simulink model "Plant"  (R2021a)
settings: Solver=ode8  StartTime=0.0  StopTime=20  FixedStep=0.0001  RelTol=1e-3
model workspace (MAT data in the model file):
  initial_current = 0
undefined symbols (not defined in the file): DiscIntNeverNeededParam
settings Model: Creator=zhaoh  LastModifiedBy=zhaoh

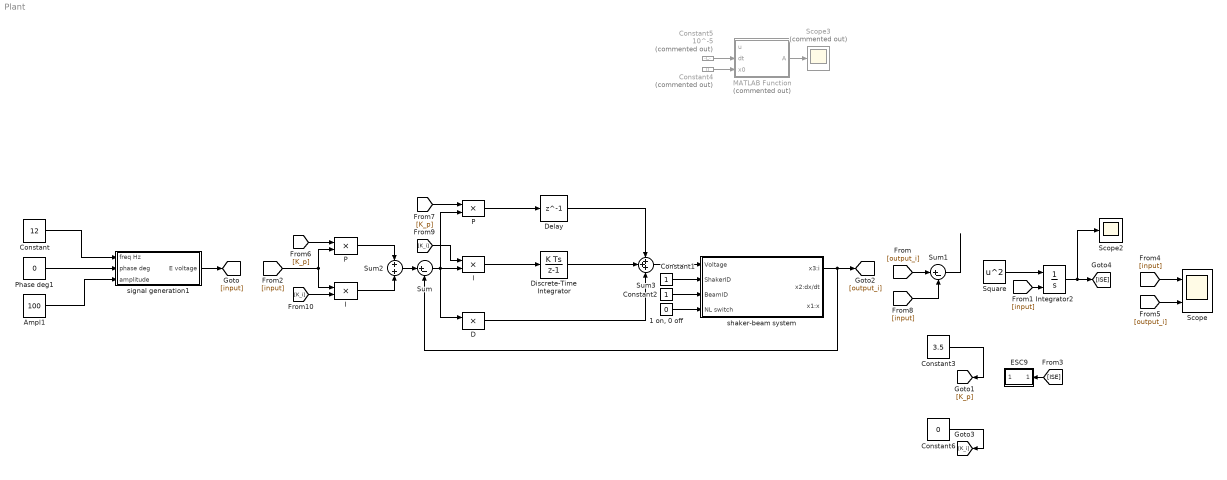
== system Plant ==
  "1 on, 0 off" : Constant  Value=0
  Ampl1 : Constant  Value=100
  Constant : Constant  Value=12
  Constant1 : Constant
  Constant2 : Constant
  Constant3 : Constant  Value=3.5
  Constant4 : Constant  Commented=on  Value=0
  Constant5 : Constant  Commented=on  Value=10^-5
  Constant6 : Constant  Value=0
  "D " : Product
  Delay : Delay  DelayLength=1
  Discrete-Time Integrator : DiscreteIntegrator  SampleTime=-1  ICPrevOutput=DiscIntNeverNeededParam  ICPrevScaledInput=DiscIntNeverNeededParam
  ESC9 : Subsystem
  I : Product
  "I " : Product
  Integrator2 : Integrator  ExternalReset=rising
  MATLAB Function : MATLAB Function  Commented=on  TreatAsAtomicUnit=on
  P : Product
  "P " : Product
  Phase deg1 : Constant  Value=0
  Scope : Scope  NumInputPorts=2
  Scope2 : Scope
  Scope3 : Scope  Commented=on
  Square : Math  Operator=square  SaturateOnIntegerOverflow=on
  Sum : Sum  Inputs=|+-
  Sum1 : Sum  Inputs=|+-
  Sum2 : Sum
  Sum3 : Sum  Inputs=+++
  shaker-beam system : Subsystem
  signal generation1 : Subsystem
  wires:
  Constant/1 -> signal generation1/1(freq Hz)
  Ampl1/1 -> signal generation1/3(amplitude)
  Phase deg1/1 -> signal generation1/2(phase deg)
  Sum3/1 -> shaker-beam system/1(Voltage)
  Constant1/1 -> shaker-beam system/2(ShakerID)
  Constant2/1 -> shaker-beam system/3(BeamID)
  "1 on, 0 off"/1 -> shaker-beam system/4(NL switch)
  Sum1/1 -> ?
  Square/1 -> Integrator2/1
  [output_i] -> Sum1/1
  [input] -> Integrator2/2
  Integrator2/1 -> Scope2/1, [ISE]
  [ISE] -> ESC9/1(out)
  [input] -> Scope/1
  [output_i] -> Scope/2
  shaker-beam system/1(x3:i) -> Sum/2, [output_i]
  [input] -> Sum1/2
  Constant4/1 -> MATLAB Function/3(x0)
  Constant5/1 -> MATLAB Function/2(dt)
  MATLAB Function/1(A) -> Scope3/1
  signal generation1/1(E voltage) -> [input]
  [input] -> I/1, P/2
  Sum2/1 -> Sum/1
  I/1 -> Sum2/2
  P/1 -> Sum2/1
  "D "/1 -> Sum3/3
  "P "/1 -> Delay/1
  "I "/1 -> Discrete-Time Integrator/1
  Sum/1 -> "D "/1, "P "/2, "I "/2
  [K_p] -> P/1
  Constant3/1 -> [K_p]
  [K_p] -> "P "/1
  [K_i] -> "I "/1
  Constant6/1 -> [K_i]
  [K_i] -> I/2
  Discrete-Time Integrator/1 -> Sum3/2
  Delay/1 -> Sum3/1

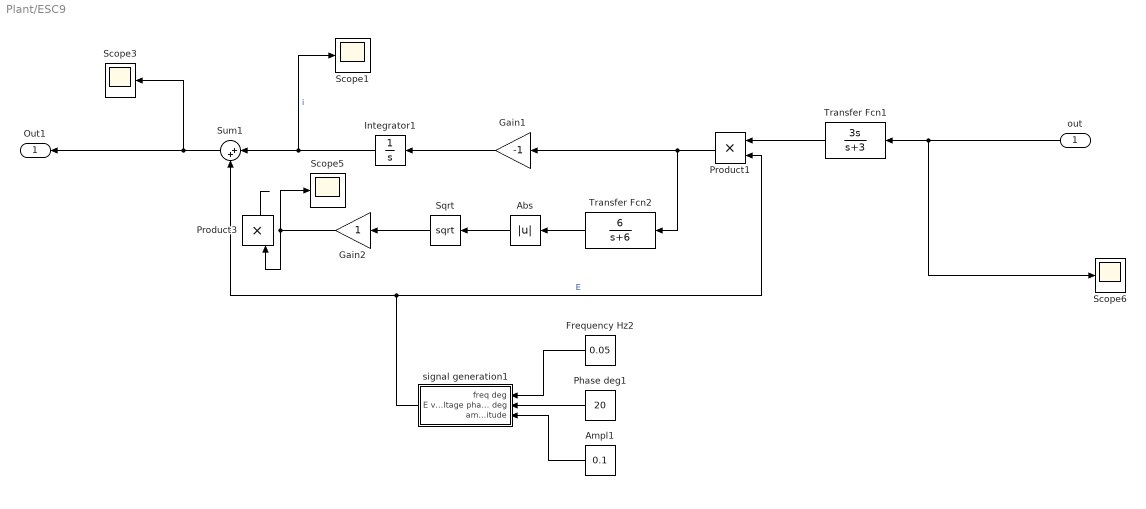
== system Plant/ESC9 ==
  out : Inport
  Abs : Abs
  Ampl1 : Constant  Value=0.1
  Frequency Hz2 : Constant  Value=0.05
  Gain1 : Gain  Gain=-1
  Gain2 : Gain
  Integrator1 : Integrator  LowerSaturationLimit=0
  Phase deg1 : Constant  Value=20
  Product1 : Product
  Product3 : Product
  Scope{1,3,5..6} (4 alike) : Scope
  Sqrt : Sqrt  SaturateOnIntegerOverflow=on
  Sum1 : Sum  Inputs=|++
  Transfer Fcn1 : TransferFcn  Numerator=[3 0]  Denominator=[1 3]
  Transfer Fcn2 : TransferFcn  Numerator=[6]  Denominator=[1 6]
  signal generation1 : Subsystem
  Out1 : Outport
  wires:
  Sum1/1 -> Scope3/1, Out1/1
  out/1 -> Scope6/1, Transfer Fcn1/1
  Transfer Fcn1/1 -> Product1/1
  Product1/1 -> Transfer Fcn2/1, Gain1/1
  Integrator1/1 -> Scope1/1, Sum1/1  "i"
  Phase deg1/1 -> signal generation1/2(phase deg)
  Ampl1/1 -> signal generation1/3(amplitude)
  Frequency Hz2/1 -> signal generation1/1(freq deg)
  signal generation1/1(E voltage) -> Sum1/2, Product1/2  "E"
  Transfer Fcn2/1 -> Abs/1
  Abs/1 -> Sqrt/1
  Product3/1 -> ?
  Sqrt/1 -> Gain2/1
  Gain2/1 -> Scope5/1, Product3/2
  Gain1/1 -> Integrator1/1

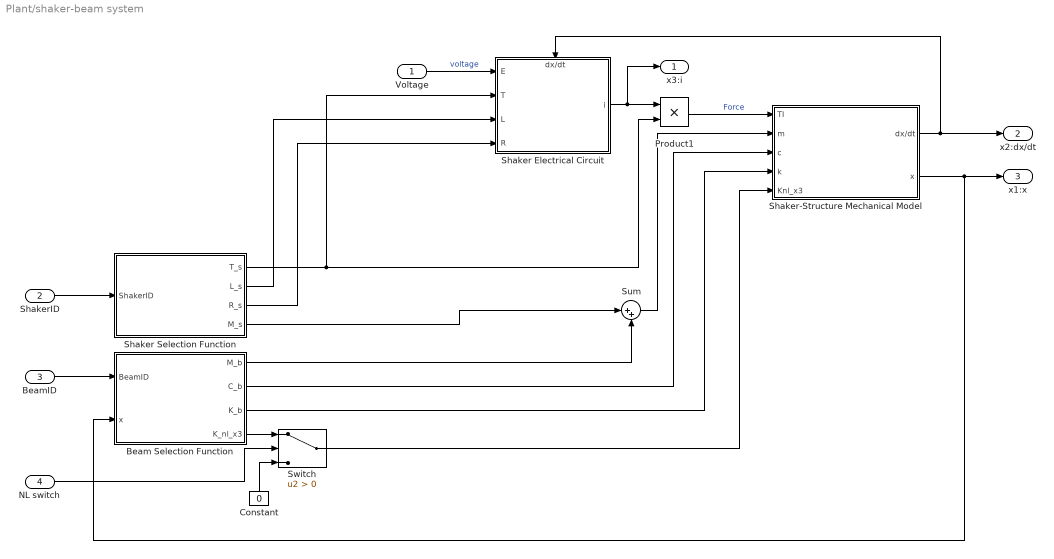
== system Plant/shaker-beam system ==
  Voltage : Inport
  ShakerID : Inport  Port=2
  BeamID : Inport  Port=3
  NL switch : Inport  Port=4
  Beam Selection Function : MATLAB Function  TreatAsAtomicUnit=on
  Constant : Constant  Value=0
  Product1 : Product
  Shaker Electrical Circuit : Subsystem
      settings: PortSchema="{\"entries\":[{\"content\":{\"sides\":[{\"content\":{\"connectorIds\":[\"In1\",\"In2\",\"In3\",\"In4\"]},\"type\":\"ConnectorPlacement.EquallySpacedRectSide\",\"uuid\":\"0d3c555b-12b6-43fe-a0ab-5f3e3cbd0fce\"},{\"content\":{\"connectorIds\":[\"Out1\"],\"side\":\"RIGHT\"},\"type\":\"ConnectorPlacement.EquallySpacedRectSide\",\"uuid\":\"7ee828ba-1fb1-406e-b6d6-19bcbb73e609\"},{\"content\":{\"connectorIds\":[\"In5\"],\"side\":\"TOP\"},\"type\":\"ConnectorPlacement.EquallySpacedRectSide\",\"uuid\":\"6ee8eddd-bc38-49cf-b56f-2a5b98a85fed\"},{\"content\":{\"connectorIds\":[],\"side\":\"BOTTOM\"},\"type\":\"ConnectorPlacement.EquallySpacedRectSide\",\"uuid\":\"38ac5a0f-1b40-47a3-ad3e-0b6df910b1ee\"}]},\"type\":\"ConnectorPlacement.EquallySpacedConnector\",\"uuid\":\"ad2dfaca-37f2-4594-907e-8526ee15e3f0\"}],\"packageUris\":[\"http://schema.mathworks.com/mf0/Connector/R2020b\"],\"version\":\"1.0\"}"
  Shaker Selection Function : MATLAB Function  TreatAsAtomicUnit=on
  Shaker-Structure Mechanical Model : Subsystem
  Sum : Sum  Inputs=|++
  Switch : Switch  Criteria=u2 > Threshold
  x3:i : Outport
  x2:dx/dt : Outport  Port=2
  x1:x : Outport  Port=3
  wires:
  Sum/1 -> Shaker-Structure Mechanical Model/2(m)
  Shaker Selection Function/3(R_s) -> Shaker Electrical Circuit/4(R)
  Beam Selection Function/2(C_b) -> Shaker-Structure Mechanical Model/3(c)
  Shaker-Structure Mechanical Model/1(dx/dt) -> x2:dx/dt/1, Shaker Electrical Circuit/5(dx/dt)
  Shaker Selection Function/1(T_s) -> Shaker Electrical Circuit/2(T), Product1/2
  Shaker Selection Function/2(L_s) -> Shaker Electrical Circuit/3(L)
  Shaker-Structure Mechanical Model/2(x) -> Beam Selection Function/2(x), x1:x/1
  Switch/1 -> Shaker-Structure Mechanical Model/5(Knl_x3)
  Shaker Selection Function/4(M_s) -> Sum/1
  Beam Selection Function/1(M_b) -> Sum/2
  Product1/1 -> Shaker-Structure Mechanical Model/1(TI)  "Force"
  Voltage/1 -> Shaker Electrical Circuit/1(E)  "voltage"
  ShakerID/1 -> Shaker Selection Function/1(ShakerID)
  BeamID/1 -> Beam Selection Function/1(BeamID)
  Shaker Electrical Circuit/1(i) -> x3:i/1, Product1/1
  NL switch/1 -> Switch/2
  Constant/1 -> Switch/3
  Beam Selection Function/4(K_nl_x3) -> Switch/1
  Beam Selection Function/3(K_b) -> Shaker-Structure Mechanical Model/4(k)

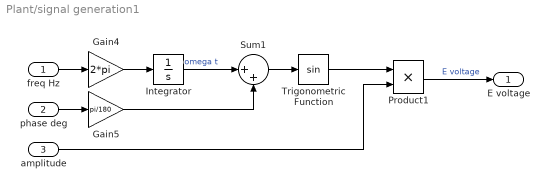
== system Plant/signal generation1 ==
  freq Hz : Inport
  phase deg : Inport  Port=2
  amplitude : Inport  Port=3
  Gain4 : Gain  Gain=2*pi
  Gain5 : Gain  Gain=pi/180
  Integrator : Integrator
  Product1 : Product
  Sum1 : Sum  Inputs=|++
  Trigonometric Function : Trigonometry
  E voltage : Outport
  wires:
  Trigonometric Function/1 -> Product1/1
  phase deg/1 -> Gain5/1
  Sum1/1 -> Trigonometric Function/1
  amplitude/1 -> Product1/2
  Product1/1 -> E voltage/1  "E voltage"
  Integrator/1 -> Sum1/1  "omega t"
  freq Hz/1 -> Gain4/1
  Gain4/1 -> Integrator/1
  Gain5/1 -> Sum1/2

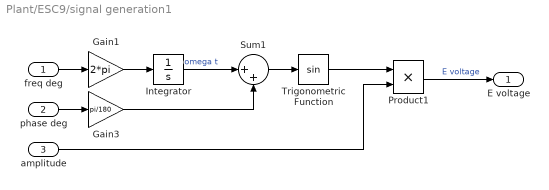
== system Plant/ESC9/signal generation1 ==
  freq deg : Inport
  phase deg : Inport  Port=2
  amplitude : Inport  Port=3
  Gain1 : Gain  Gain=2*pi
  Gain3 : Gain  Gain=pi/180
  Integrator : Integrator
  Product1 : Product
  Sum1 : Sum  Inputs=|++
  Trigonometric Function : Trigonometry
  E voltage : Outport
  wires:
  Gain3/1 -> Sum1/2
  phase deg/1 -> Gain3/1
  Gain1/1 -> Integrator/1
  freq deg/1 -> Gain1/1
  Integrator/1 -> Sum1/1  "omega t"
  Product1/1 -> E voltage/1  "E voltage"
  amplitude/1 -> Product1/2
  Sum1/1 -> Trigonometric Function/1
  Trigonometric Function/1 -> Product1/1

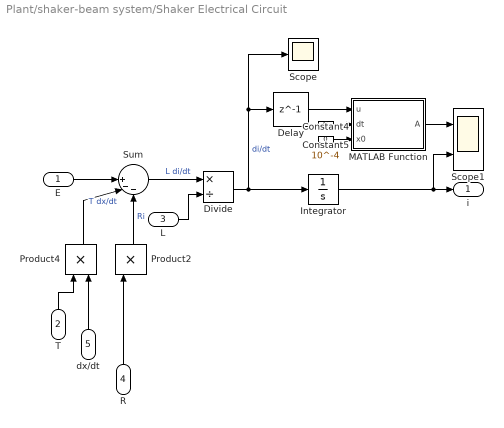
== system Plant/shaker-beam system/Shaker Electrical Circuit ==
  E : Inport
  T : Inport  Port=2
  L : Inport  Port=3
  R : Inport  Port=4
  dx/dt : Inport  Port=5
  Constant4 : Constant  Value=0
  Constant5 : Constant  Value=10^-4
  Delay : Delay  DelayLength=1
  Divide : Product  Inputs=*/
  Integrator : Integrator
  MATLAB Function : MATLAB Function  TreatAsAtomicUnit=on
  Product2 : Product
  Product4 : Product
  Scope : Scope
  Scope1 : Scope  NumInputPorts=2
  Sum : Sum  Inputs=||+--
  i : Outport
  wires:
  R/1 -> Product2/1
  Product2/1 -> Sum/3  "Ri"
  L/1 -> Divide/2
  Sum/1 -> Divide/1  "L di/dt"
  Divide/1 -> Integrator/1, Delay/1, Scope/1  "di/dt"
  Product4/1 -> Sum/2  "T dx/dt"
  dx/dt/1 -> Product4/2
  T/1 -> Product4/1
  E/1 -> Sum/1
  Constant4/1 -> MATLAB Function/3(x0)
  Constant5/1 -> MATLAB Function/2(dt)
  Integrator/1 -> Scope1/2, i/1
  Delay/1 -> MATLAB Function/1(u)
  MATLAB Function/1(A) -> Scope1/1

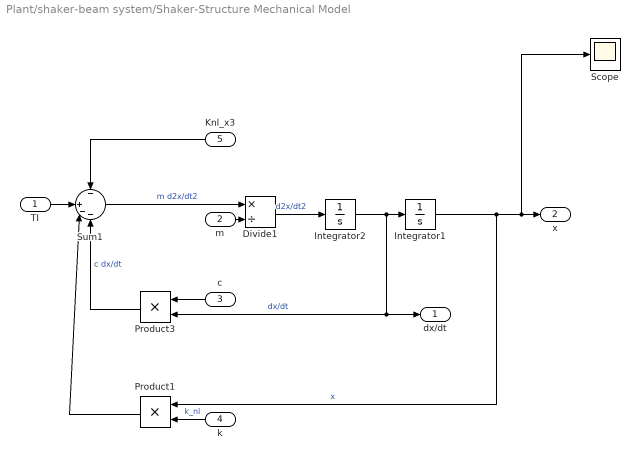
== system Plant/shaker-beam system/Shaker-Structure Mechanical Model ==
  TI : Inport
  m : Inport  Port=2
  c : Inport  Port=3
  k : Inport  Port=4
  Knl_x3 : Inport  Port=5
  Divide1 : Product  Inputs=*/
  Integrator1 : Integrator
  Integrator2 : Integrator
  Product1 : Product
  Product3 : Product
  Scope : Scope
  Sum1 : Sum  Inputs=-|+--
  dx/dt : Outport
  x : Outport  Port=2
  wires:
  m/1 -> Divide1/2
  Divide1/1 -> Integrator2/1  "d2x/dt2"
  Sum1/1 -> Divide1/1  "m d2x/dt2"
  Product3/1 -> Sum1/4  "c dx/dt"
  Knl_x3/1 -> Sum1/1
  c/1 -> Product3/1
  Integrator1/1 -> Scope/1, x/1, Product1/1  "x"
  TI/1 -> Sum1/2
  k/1 -> Product1/2  "k_nl"
  Product1/1 -> Sum1/3
  Integrator2/1 -> dx/dt/1, Product3/2, Integrator1/1  "dx/dt"

== matlab function Plant/shaker-beam system/Beam Selection Function ==
  data: BeamID input; M_b output; C_b output; K_b output; K_nl_x3 output; x input
function [M_b, C_b, K_b, K_nl_x3] = fcn(BeamID, x)
if BeamID == 1 % beam data from A.D.Shaw - 2016 - Periodic responses of a structure with 3 to 1 internal resonance
    M_b = 0.04;
    C_b = 0.044;
    K_b = 121;
    K_nl = 2.967*10^6; 
    elseif BeamID == 2 % beam data made up
    M_b = 0.03;
    C_b = 0.022;
    K_b = 15;
    K_nl = 1.845*10^6; 
else % unvalid shaker id
    M_b = 0;
    C_b = 0;
    K_b = 0;
    K_nl = 0; 
    disp('error');
end 
K_nl_x3 = K_nl*x^3;
end

== matlab function Plant/shaker-beam system/Shaker Selection Function ==
  data: ShakerID input; T_s output; L_s output; R_s output; M_s output
function [T_s, L_s, R_s, M_s]= fcn(ShakerID)
%% uncomment this section for proposed system and normal operation
if ShakerID == 1 % shaker data from Benjamin R 2021 - Shaker-structure interaction modeling and analysis for nonlinear force appropriation testing
    T_s = 18.5; % = BL 
    L_s = 1*10^(-5); 
    R_s = 6.6;
    M_s = 0.037+0.136; % = m_2 + m_3
%% do not uncomment this section unless you want to check for mahdi's shaker model
% if ShakerID == 1 % shaker data from Mahdi Bzeih - 2017 - Large scale shaker emulator
%     T_s = 1.782; % = N*B*l_c
%     L_s = 4.058*10^(-5);
%     R_s = 0.135;
%     M_s = 2+4.4; % = m_2 + m_3
%% do the section normally and those commenting shit ends here
    elseif ShakerID == 2 % shaker data made up
    T_s = 10;
    L_s = 1.3*10^(5);
    R_s = 8.6;
    M_s = 0.047;
else % unvalid shaker id
    T_s = 0;
    L_s = 0;
    R_s = 0;
    M_s = 0; 
    disp('error');
end 
end

== matlab function Plant/MATLAB Function ==
  data: u input; A output; dt input; x0 input
function A = fcn(u, dt, x0)
%define input at previous step
persistent ud
    if isempty(ud)
        ud = 0;
    end
%calculate increment of integral
dA = (u+ud)*dt/2;
%define integration at previous step
persistent Ad
    %specify initial condition
    if isempty(Ad)
        Ad = x0;
    end
%calculate integration
A = Ad + dA;
%update previous step parameters
Ad = A;
ud = u;

== matlab function Plant/shaker-beam system/Shaker Electrical Circuit/MATLAB Function ==
  settings: updateMethod=DISCRETE
  data: u input; A output; dt input; x0 input
function A = fcn(u, dt, x0)
%define input at previous step
persistent ud
    if isempty(ud)
        ud = 0;
    end
%calculate increment of integral
dA = (u+ud)*dt/2;
%define integration at previous step
persistent Ad
    %specify initial condition
    if isempty(Ad)
        Ad = x0;
    end
%calculate integration
A = Ad + dA;
%update previous step parameters
Ad = A;
ud = u;
